simulink model "CTRL_test"  (R2024b)
settings: Solver=VariableStepAuto  StartTime=0.0  StopTime=10.0  RelTol=1e-3
libraries: CTRL x1
settings Model: Creator=blatak  LastModifiedBy=blatak

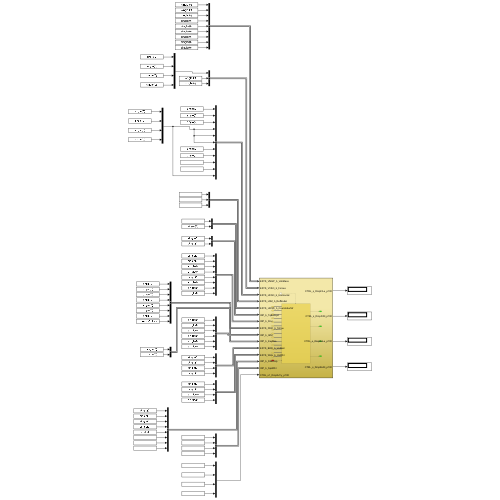
[thumbnail: Simulink's stored preview of the top-level diagram]
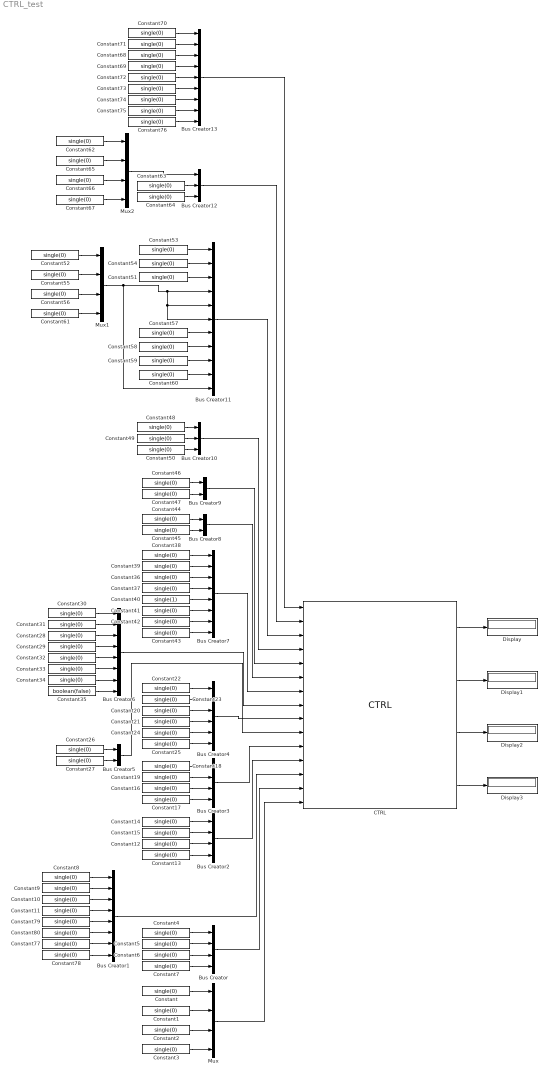
== system CTRL_test ==
  Bus Creator : BusCreator  Inputs=4  OutDataTypeStr=Bus: INP_b_SpdWhl
      settings: InheritFromInputs=off
  Bus Creator1 : BusCreator  Inputs=8  OutDataTypeStr=Bus: INP_b_StrkDmp
      settings: InheritFromInputs=off
  Bus Creator10 : BusCreator  Inputs=3  OutDataTypeStr=Bus: ESTS_LSM_b_RefModel
      settings: InheritFromInputs=off
  Bus Creator11 : BusCreator  Inputs=11  OutDataTypeStr=Bus: ESTS_VHSO_b_Horizontal
      settings: InheritFromInputs=off
  Bus Creator12 : BusCreator  Inputs=3  OutDataTypeStr=Bus: ESTS_VVSO_b_Forces
      settings: InheritFromInputs=off
  Bus Creator13 : BusCreator  Inputs=9  OutDataTypeStr=Bus: ESTS_VMGP_b_VehMass
      settings: InheritFromInputs=off
  Bus Creator2 : BusCreator  Inputs=4  OutDataTypeStr=Bus: ESTS_b_VelWhl
      settings: InheritFromInputs=off
  Bus Creator3 : BusCreator  Inputs=4  OutDataTypeStr=Bus: ESTS_b_VelBod
      settings: InheritFromInputs=off
  Bus Creator4 : BusCreator  Inputs=6  OutDataTypeStr=Bus: INP_b_IMU
      settings: InheritFromInputs=off
  Bus Creator5 : BusCreator  Inputs=2  OutDataTypeStr=Bus: INP_b_KeyBoa
      settings: InheritFromInputs=off
  Bus Creator6 : BusCreator  Inputs=8  OutDataTypeStr=Bus: ESTS_FRIC_b_friCoe
      settings: InheritFromInputs=off
  Bus Creator7 : BusCreator  Inputs=8  OutDataTypeStr=Bus: INP_b_Drvr
      settings: InheritFromInputs=off
  Bus Creator8 : BusCreator  Inputs=2  OutDataTypeStr=Bus: INP_b_TqBrkHyd
      settings: InheritFromInputs=off
  Bus Creator9 : BusCreator  Inputs=2  OutDataTypeStr=Bus: ESTS_UOD_b_OverUnderStr
      settings: InheritFromInputs=off
  CTRL : CTRL/CTRL  SystemSampleTime=-1  VariantActivationTime=update diagram  AllowFlexibleInterface=on  Latency=0  AutoFrameSizeCalculation=off
  Constant{,1..34,36..39,41..80} (79 alike) : Constant  Value=single(0)
  Constant35 : Constant  Value=boolean(false)
  Constant40 : Constant  Value=single(1)
  Display{,1..3} (4 alike) : Display
  Mux : Mux
  Mux1 : Mux
  Mux2 : Mux
  wires:
  Constant60/1 -> Bus Creator11/10
  Constant7/1 -> Bus Creator/4
  Bus Creator/1 -> CTRL/14
  Bus Creator4/1 -> CTRL/9
  Bus Creator12/1 -> CTRL/2
  Constant6/1 -> Bus Creator/3
  Constant3/1 -> Mux/4
  Mux/1 -> CTRL/15
  Constant12/1 -> Bus Creator2/3
  Constant15/1 -> Bus Creator2/2
  Constant13/1 -> Bus Creator2/4
  Constant14/1 -> Bus Creator2/1
  Constant63/1 -> Bus Creator12/2
  Constant64/1 -> Bus Creator12/3
  Constant8/1 -> Bus Creator1/1
  Constant9/1 -> Bus Creator1/2
  Constant11/1 -> Bus Creator1/4
  Constant10/1 -> Bus Creator1/3
  Constant30/1 -> Bus Creator6/1
  Constant31/1 -> Bus Creator6/2
  Constant33/1 -> Bus Creator6/6
  Constant28/1 -> Bus Creator6/3
  Constant29/1 -> Bus Creator6/4
  Constant5/1 -> Bus Creator/2
  Constant59/1 -> Bus Creator11/9
  Constant2/1 -> Mux/3
  Constant/1 -> Mux/1
  Constant34/1 -> Bus Creator6/7
  Constant1/1 -> Mux/2
  Bus Creator11/1 -> CTRL/3
  Constant56/1 -> Mux1/3
  Constant55/1 -> Mux1/2
  Constant52/1 -> Mux1/1
  Constant61/1 -> Mux1/4
  Constant54/1 -> Bus Creator11/2
  Constant32/1 -> Bus Creator6/5
  Constant53/1 -> Bus Creator11/1
  Constant51/1 -> Bus Creator11/3
  Bus Creator10/1 -> CTRL/4
  Constant26/1 -> Bus Creator5/1
  Constant65/1 -> Mux2/2
  Constant67/1 -> Mux2/4
  Bus Creator3/1 -> CTRL/11
  Constant72/1 -> Bus Creator13/5
  Constant74/1 -> Bus Creator13/7
  Constant68/1 -> Bus Creator13/3
  Constant70/1 -> Bus Creator13/1
  Constant71/1 -> Bus Creator13/2
  Constant62/1 -> Mux2/1
  Bus Creator5/1 -> CTRL/10
  Constant48/1 -> Bus Creator10/1
  Constant49/1 -> Bus Creator10/2
  Constant16/1 -> Bus Creator3/3
  Constant18/1 -> Bus Creator3/1
  Constant73/1 -> Bus Creator13/6
  Constant17/1 -> Bus Creator3/4
  Mux2/1 -> Bus Creator12/1
  Bus Creator8/1 -> CTRL/6
  Constant19/1 -> Bus Creator3/2
  Constant46/1 -> Bus Creator9/1
  Constant47/1 -> Bus Creator9/2
  Constant25/1 -> Bus Creator4/6
  Bus Creator1/1 -> CTRL/13
  Bus Creator9/1 -> CTRL/5
  Constant57/1 -> Bus Creator11/7
  Constant4/1 -> Bus Creator/1
  Constant44/1 -> Bus Creator8/1
  Constant36/1 -> Bus Creator7/3
  Constant50/1 -> Bus Creator10/3
  Constant66/1 -> Mux2/3
  Constant38/1 -> Bus Creator7/1
  Constant42/1 -> Bus Creator7/7
  Constant24/1 -> Bus Creator4/5
  Constant37/1 -> Bus Creator7/4
  Constant39/1 -> Bus Creator7/2
  Constant69/1 -> Bus Creator13/4
  Constant40/1 -> Bus Creator7/5
  Constant43/1 -> Bus Creator7/8
  Constant27/1 -> Bus Creator5/2
  Bus Creator6/1 -> CTRL/8
  Constant23/1 -> Bus Creator4/2
  Bus Creator2/1 -> CTRL/12
  Constant22/1 -> Bus Creator4/1
  Constant41/1 -> Bus Creator7/6
  Bus Creator7/1 -> CTRL/7
  Constant20/1 -> Bus Creator4/3
  Constant58/1 -> Bus Creator11/8
  Mux1/1 -> Bus Creator11/11, Bus Creator11/6, Bus Creator11/5, Bus Creator11/4
  Bus Creator13/1 -> CTRL/1
  Constant75/1 -> Bus Creator13/8
  Constant35/1 -> Bus Creator6/8
  Constant76/1 -> Bus Creator13/9
  Constant21/1 -> Bus Creator4/4
  Constant45/1 -> Bus Creator8/2
  CTRL/1 -> Display/1
  CTRL/2 -> Display1/1
  CTRL/3 -> Display2/1
  CTRL/4 -> Display3/1
  Constant78/1 -> Bus Creator1/8
  Constant77/1 -> Bus Creator1/7
  Constant80/1 -> Bus Creator1/6
  Constant79/1 -> Bus Creator1/5
